simulink model "astron_hw_test_au50_16k_8in"  (R2021a)
settings: Solver=VariableStepDiscrete  StartTime=0.0  StopTime=32000  RelTol=1e-3
undefined symbols (not defined in the file): d0, d1, d2, d3, d4, d5, d6, d7, FFT, sr, Wideband_FFT
libraries: xbsIndex_r4 x1247, casper_library_misc x6, xps_library x1
(part 4 of 17)

== system astron_hw_test_au50_16k_8in/bram_in4 ==
  addr : Inport
  data_in : Inport  Port=2
  we : Inport  Port=3
  Terminator : Terminator
  Terminator1 : Terminator
  Terminator2 : Terminator
  astron_hw_test_au50_16k_8in_bram_in4_addr : xbsIndex_r4/Gateway Out  inherit_from_input=off  hdl_port=on  rows=1  columns=1  UseAsDAC=off  DACChannel='1'  interface=None  automatic_assignment=on  address_offset=hex2dec('00')  intf_name=''  intf_description=''  timing_constraint=None  locs_specified=off  LOCs={'A5','B9','A9','C1','A3','G6','E9','A6','A7','A8','B8','B1','B3','D9','B5','B4','B6','C2'}  io_standard={}  block_type=gatewayout
      settings: infoedit="Gateway out block.  Converts Xilinx fixed point inputs into ouputs of type Simulink integer, double, or fixed point.<P><P>Hardware notes:  In hardware these blocks become top level output ports or are discarded, depending on how they are configured."  sginterface={'Nallatech'=>{'xdspkit'=>{'non_memory_mapped_port'=>'uprev_Shared_BRAM_addr'}},'Xilinx'=>{'jtaghwcosim'=>{'non_memory_mapped_port'=>'uprev_Shared_BRAM_addr'},'xdspkit'=>{'non_memory_mapped_port'=>'uprev_Shared_BRAM_addr'}}}  xl_area=[0, 0, 0, 0, 0, 0, 0]
  astron_hw_test_au50_16k_8in_bram_in4_data_in : xbsIndex_r4/Gateway Out  inherit_from_input=off  hdl_port=on  rows=1  columns=1  UseAsDAC=off  DACChannel='1'  interface=None  automatic_assignment=on  address_offset=hex2dec('00')  intf_name=''  intf_description=''  timing_constraint=None  locs_specified=off  LOCs={'B21','B22','A22','B23','B19','C19','A20','A21','A23','B24','A24','A25','E18','D18','C18','B18'}  io_standard={}  block_type=gatewayout
      settings: infoedit="Gateway out block.  Converts Xilinx fixed point inputs into ouputs of type Simulink integer, double, or fixed point.<P><P>Hardware notes:  In hardware these blocks become top level output ports or are discarded, depending on how they are configured."  sginterface={'Nallatech'=>{'xdspkit'=>{'non_memory_mapped_port'=>'uprev_Shared_BRAM_data_in'}},'Xilinx'=>{'jtaghwcosim'=>{'non_memory_mapped_port'=>'uprev_Shared_BRAM_data_in'},'xdspkit'=>{'non_memory_mapped_port'=>'uprev_Shared_BRAM_data_in'}}}  xl_area=[0, 0, 0, 0, 0, 0, 0]
  astron_hw_test_au50_16k_8in_bram_in4_data_out : xbsIndex_r4/Gateway In  gui_display_data_type=Fixed-point  arith_type=Unsigned  n_bits=32  bin_pt=0  preci_type=Single  exp_width=8  frac_width=24  rows=1  columns=1  quantization=Truncate  overflow=Wrap  period=sample_rate  UseAsADC=off  ADCChannel='1'  interface=None  automatic_assignment=on  address_offset=hex2dec('00')  intf_name=''  intf_description=''  default_value=0  timing_constraint=None  locs_specified=off  LOCs={}  io_standard={}  inherit_from_input=off  hdl_port=on  dbl_ovrd=off  block_type=gatewayin
      settings: xl_area=[0, 0, 0, 0, 0, 0, 0]
  astron_hw_test_au50_16k_8in_bram_in4_we : xbsIndex_r4/Gateway Out  inherit_from_input=off  hdl_port=on  rows=1  columns=1  UseAsDAC=off  DACChannel='1'  interface=None  automatic_assignment=on  address_offset=hex2dec('00')  intf_name=''  intf_description=''  timing_constraint=None  locs_specified=off  LOCs={'A14'}  io_standard={}  block_type=gatewayout
      settings: infoedit="Gateway out block.  Converts Xilinx fixed point inputs into ouputs of type Simulink integer, double, or fixed point.<P><P>Hardware notes:  In hardware these blocks become top level output ports or are discarded, depending on how they are configured."  xl_area=[0, 0, 0, 0, 0, 0, 0]
  calc_add : Subsystem  mask{data_width=32, addr_width=11, sample_rate=sample_rate}
      mask prompts: data_width "data width"; addr_width "address width"; sample_rate "sample rate"
  convert_addr : xbsIndex_r4/Convert  gui_display_data_type=Fixed-point  arith_type=Unsigned  n_bits=addr_width  bin_pt=0  float_type=Single  exp_bits=8  fraction_bits=24  quantization=Truncate  overflow=Wrap  en=off  latency=0  pipeline=off  dbl_ovrd=off  block_type=convert
      settings: xl_area=[0, 0, 0, 0, 0, 0, 0]
  convert_din1 : xbsIndex_r4/Convert  gui_display_data_type=Fixed-point  arith_type=Unsigned  n_bits=32  bin_pt=0  float_type=Single  exp_bits=8  fraction_bits=24  quantization=Truncate  overflow=Wrap  en=off  latency=0  pipeline=off  dbl_ovrd=off  block_type=convert
      settings: xl_area=[0, 0, 0, 0, 0, 0, 0]
  convert_we : xbsIndex_r4/Convert  gui_display_data_type=Fixed-point  arith_type=Unsigned  n_bits=1  bin_pt=0  float_type=Single  exp_bits=8  fraction_bits=24  quantization=Truncate  overflow=Wrap  en=off  latency=0  pipeline=off  dbl_ovrd=off  block_type=convert
      settings: xl_area=[0, 0, 0, 0, 0, 0, 0]
  munge_in : Subsystem  AncestorBlock=casper_library_flow_control/munge  mask(munge){divisions=1, div_size=32, order=[0], arith_type_out=Unsigned, bin_pt_out=0}
      mask prompts: divisions "Number of divisions"; div_size "Division size (bits)"; order "Division packing order"; arith_type_out "Output arithmetic type"; bin_pt_out "Output binary point"
      mask help: Splits an input bus into the specified number of divisions and then recombines them in the order specified (most significant division = 0,least = number divisions-1)
      mask init:
      | munge_init(gcb, ...
      |     'divisions', divisions, ...
      |     'div_size', div_size, ...
      |     'order', order, ...
      |     'arith_type_out', arith_type_out, ...
      |     'bin_pt_out', bin_pt_out);
      settings: AttributesFormatString=|
      | split:32
      | join:0
      | Unsigned [32,0]
      mask TypeOptions arith_type_out: Unsigned | Signed  (2's comp) | Floating-point
  munge_out : Subsystem  AncestorBlock=casper_library_flow_control/munge  mask(munge){divisions=1, div_size=32, order=[0], arith_type_out=Signed  (2's comp), bin_pt_out=0}
      mask prompts: divisions "Number of divisions"; div_size "Division size (bits)"; order "Division packing order"; arith_type_out "Output arithmetic type"; bin_pt_out "Output binary point"
      mask help: Splits an input bus into the specified number of divisions and then recombines them in the order specified (most significant division = 0,least = number divisions-1)
      mask init:
      | munge_init(gcb, ...
      |     'divisions', divisions, ...
      |     'div_size', div_size, ...
      |     'order', order, ...
      |     'arith_type_out', arith_type_out, ...
      |     'bin_pt_out', bin_pt_out);
      settings: AttributesFormatString=|
      | split:32
      | join:0
      | Signed  (2's comp) [32,0]
      mask TypeOptions arith_type_out: Unsigned | Signed  (2's comp) | Floating-point
  sim_mem : Subsystem  mask{arith_type=Signed  (2's comp), addr_width=11, data_width=32, data_bin_pt=0, init_vals=[5372    264   2664  -1583   -209  -8118   2914  -1119   9156  -1791   -682  -1639  -1972  -7418   7738  -6315   6175   2047  -1371  -5922   1133  -4748   4947  -7294    598    694  -2771 -11240  -7297  -1257  10652  -4301    242  -5536  -2316  -5035   -774 -11427   5804  -3502  -2727  -5631   5820  -1336   3152    207   3505  -2899   3712  -5832   -548    499   -949    356   4168  -2711   9110  -1446   -185  -7623   5256   -721  -2371   1834  -3171  -2617  -2004  -5374   8059  -8009   3468  -4248   6229  -5263   7567    392  -2288  -3689   -834   3206   -427   2199   3578  -3080   7720  -4480  -1270  -1827    789  -3782   2421   3593    783   3234  10007  -5331  -3342   3673   3588    706   4326  -4419   -132  -6818   2728  -1544   2912  -6007  -4264  -5624   8559  -4103  -1178   -386   2151  -2551  -1873   3145   1273  -4488  -2723    612   -822  -5199   4364   8473   5041   1818  -1070  -2280   3607  -3180   7444  -4879   6916  -2006   5554  -3584    161   3913   6382   1474   -131  -6736  -3432   1085   3615   -949    406  -3710  10859   -234   3318  -8376   4924   6284  -1230  -6191   2438   1240  -1100  -7300   6874  -1202  -3786   -162  -3936  -1656   3000  -2820   2006  -1797  -4165  -1961   3081  -2189   2194  -5197   5790   2148   1526 -12939   4539   2170   -302  -8231   4511  -4644  -2325  -1395  -2217  -5029   -259    343   4026  11402   9172    170   3063   7245   2744   2974   -116   2113   5449   -744   1639  -8436   2860   7361   -750  -2950   5828   4070   4301  -3510  -3373    239   6919   5964   -550  -3159   2494  -2931   3776  -2781  -1672    540  11327   3666   7426  -7651   2220  -4925   5619   -307   7830  -8896   3110  -7112   8450   -647   5009  -4269   1593  -3851   1861    757   3866    346    -32  -6926  -2968   -124   2070  -6109  -1641 -12060  -1216  -2148  -3305   3381  -8059   -991   5600    890   -676  -8576   6527  -2235   6327  -1480  -2544  -3362  -3643    176  -2266  -4719   5604   1756  10810  -3044    204  -3243   5925   9325  11724   -278    787   1475    253  -2705   1253  -6883   4739    492   2583   4196   -702    919   4520   2806   -557   -919   6700    429   1604  -5668   5381  -5403  -4298   3048   1914   1868   -221  -1599   1680   -408   4556  -2677    531  -3197  10488  -1424   7178  -8210   1200 -10397  -1686  -6020   7446  -3039   6340     44  -2611   6013    813  -6576  -5465   2793   7907  -2877   2051  -3612   2879   -858    -20   -343   5516  -3239    276  -6001   7400  -4314  -1066  -1650   2581  -7150   7801  -5366   2259  -3747  -1802  -3143  -4562   -217   2213  -3598    380   1819    459 -11485   1496   3375   5261  -4536   2628  -4517   2812  -2382   2159   2459   1499   -603  -3458  -6213  -1555  -9169  -7572   3950   1325   -737    293    352   5860  -4078   3580  -3457  -2420   3374   5013   2542   1417  -2648    639   2635  -1587  -7108   1615  -6830  -1268  -3826  -7575  -3513   9379  -1148  -1833  -4949    799  -1823     85   2797   4700   1680   5387  -8986  -2486    672   4069  -2791   4382  -4512  -5528  -4235  -7648  -8826   5712   2253    420   4054  -1483  -3200  -1126  -3146  -4911  -8683  -6029    797   6606  -7828  -3268    594  -4858   6717   -412   2169   4283  -2812   1675   2976    658    -72   3034  -4769   3257   1926  -4680  -2421   9476  -1206   2513   4604   7309  -3175  -1675   -869   4580   3774   6399    313  -1949   -886  -2670   3019   5781  -4535   2075   2994    445  -7441   1585  -5266   2359  -7332   2614    880   1385  -2791    426  -2620   2687   1016   3193   1554   3871  -5678   3982    709   3608   6326   6781  -2259   7111  -3020    309   -524  -5932   5448   1493  -2473    647  -3940  -6107    978   2317   3384   6445   2742  -1063  -1003   3804  -2802  -9392    840    253  -2545  -1521    886   -283  -5068   3741   1149   5145  -6183   -177  -1297   6951  -1706   5403  -2825  -1015   -519  -5040 -13537  -2391  -4401  11546  -1835   3685  -5829  -2937 -12387   3257    296   5361  -2724   3034  -4443   -152   4231   3085 ...(+10338 chars)], sample_rate=1, csp_latency=1}
      mask prompts: arith_type "Output Data Type"; addr_width "Address width"; data_width "Data width"; data_bin_pt "Data Binary Point"; init_vals "Initial values"; sample_rate "Sample rate"; csp_latency "Latency"
      mask init:
      | % set_param([gcb, '/data_to_xilinx'], 'arith_type', arith_type)
      | % set_param([gcb, '/data_to_xilinx'], 'n_bits', get_param(gcb, 'data_width'))
      mask TypeOptions arith_type: Unsigned | Signed  (2's comp)
      mask TypeOptions data_width: 8 | 16 | 32 | 64 | 128
  data_out : Outport  VectorParamsAs1DForOutWhenUnconnected=off
  wires:
  munge_out/1(dout) -> data_out/1
  sim_mem/1(data_out) -> astron_hw_test_au50_16k_8in_bram_in4_data_out/1
  astron_hw_test_au50_16k_8in_bram_in4_data_out/1 -> munge_out/1(din)
  convert_addr/1 -> astron_hw_test_au50_16k_8in_bram_in4_addr/1
  convert_din1/1 -> astron_hw_test_au50_16k_8in_bram_in4_data_in/1
  data_in/1 -> munge_in/1(din)
  calc_add/1(out) -> convert_addr/1
  astron_hw_test_au50_16k_8in_bram_in4_we/1 -> Terminator2/1
  astron_hw_test_au50_16k_8in_bram_in4_data_in/1 -> Terminator1/1
  astron_hw_test_au50_16k_8in_bram_in4_addr/1 -> Terminator/1
  convert_we/1 -> astron_hw_test_au50_16k_8in_bram_in4_we/1
  addr/1 -> sim_mem/1(addr), calc_add/1(in)
  we/1 -> sim_mem/3(we), convert_we/1
  munge_in/1(dout) -> sim_mem/2(data), convert_din1/1

== system astron_hw_test_au50_16k_8in/bram_in5 ==
  addr : Inport
  data_in : Inport  Port=2
  we : Inport  Port=3
  Terminator : Terminator
  Terminator1 : Terminator
  Terminator2 : Terminator
  astron_hw_test_au50_16k_8in_bram_in5_addr : xbsIndex_r4/Gateway Out  inherit_from_input=off  hdl_port=on  rows=1  columns=1  UseAsDAC=off  DACChannel='1'  interface=None  automatic_assignment=on  address_offset=hex2dec('00')  intf_name=''  intf_description=''  timing_constraint=None  locs_specified=off  LOCs={'A5','B9','A9','C1','A3','G6','E9','A6','A7','A8','B8','B1','B3','D9','B5','B4','B6','C2'}  io_standard={}  block_type=gatewayout
      settings: infoedit="Gateway out block.  Converts Xilinx fixed point inputs into ouputs of type Simulink integer, double, or fixed point.<P><P>Hardware notes:  In hardware these blocks become top level output ports or are discarded, depending on how they are configured."  sginterface={'Nallatech'=>{'xdspkit'=>{'non_memory_mapped_port'=>'uprev_Shared_BRAM_addr'}},'Xilinx'=>{'jtaghwcosim'=>{'non_memory_mapped_port'=>'uprev_Shared_BRAM_addr'},'xdspkit'=>{'non_memory_mapped_port'=>'uprev_Shared_BRAM_addr'}}}  xl_area=[0, 0, 0, 0, 0, 0, 0]
  astron_hw_test_au50_16k_8in_bram_in5_data_in : xbsIndex_r4/Gateway Out  inherit_from_input=off  hdl_port=on  rows=1  columns=1  UseAsDAC=off  DACChannel='1'  interface=None  automatic_assignment=on  address_offset=hex2dec('00')  intf_name=''  intf_description=''  timing_constraint=None  locs_specified=off  LOCs={'B21','B22','A22','B23','B19','C19','A20','A21','A23','B24','A24','A25','E18','D18','C18','B18'}  io_standard={}  block_type=gatewayout
      settings: infoedit="Gateway out block.  Converts Xilinx fixed point inputs into ouputs of type Simulink integer, double, or fixed point.<P><P>Hardware notes:  In hardware these blocks become top level output ports or are discarded, depending on how they are configured."  sginterface={'Nallatech'=>{'xdspkit'=>{'non_memory_mapped_port'=>'uprev_Shared_BRAM_data_in'}},'Xilinx'=>{'jtaghwcosim'=>{'non_memory_mapped_port'=>'uprev_Shared_BRAM_data_in'},'xdspkit'=>{'non_memory_mapped_port'=>'uprev_Shared_BRAM_data_in'}}}  xl_area=[0, 0, 0, 0, 0, 0, 0]
  astron_hw_test_au50_16k_8in_bram_in5_data_out : xbsIndex_r4/Gateway In  gui_display_data_type=Fixed-point  arith_type=Unsigned  n_bits=32  bin_pt=0  preci_type=Single  exp_width=8  frac_width=24  rows=1  columns=1  quantization=Truncate  overflow=Wrap  period=sample_rate  UseAsADC=off  ADCChannel='1'  interface=None  automatic_assignment=on  address_offset=hex2dec('00')  intf_name=''  intf_description=''  default_value=0  timing_constraint=None  locs_specified=off  LOCs={}  io_standard={}  inherit_from_input=off  hdl_port=on  dbl_ovrd=off  block_type=gatewayin
      settings: xl_area=[0, 0, 0, 0, 0, 0, 0]
  astron_hw_test_au50_16k_8in_bram_in5_we : xbsIndex_r4/Gateway Out  inherit_from_input=off  hdl_port=on  rows=1  columns=1  UseAsDAC=off  DACChannel='1'  interface=None  automatic_assignment=on  address_offset=hex2dec('00')  intf_name=''  intf_description=''  timing_constraint=None  locs_specified=off  LOCs={'A14'}  io_standard={}  block_type=gatewayout
      settings: infoedit="Gateway out block.  Converts Xilinx fixed point inputs into ouputs of type Simulink integer, double, or fixed point.<P><P>Hardware notes:  In hardware these blocks become top level output ports or are discarded, depending on how they are configured."  xl_area=[0, 0, 0, 0, 0, 0, 0]
  calc_add : Subsystem  mask{data_width=32, addr_width=11, sample_rate=sample_rate}
      mask prompts: data_width "data width"; addr_width "address width"; sample_rate "sample rate"
  convert_addr : xbsIndex_r4/Convert  gui_display_data_type=Fixed-point  arith_type=Unsigned  n_bits=addr_width  bin_pt=0  float_type=Single  exp_bits=8  fraction_bits=24  quantization=Truncate  overflow=Wrap  en=off  latency=0  pipeline=off  dbl_ovrd=off  block_type=convert
      settings: xl_area=[0, 0, 0, 0, 0, 0, 0]
  convert_din1 : xbsIndex_r4/Convert  gui_display_data_type=Fixed-point  arith_type=Unsigned  n_bits=32  bin_pt=0  float_type=Single  exp_bits=8  fraction_bits=24  quantization=Truncate  overflow=Wrap  en=off  latency=0  pipeline=off  dbl_ovrd=off  block_type=convert
      settings: xl_area=[0, 0, 0, 0, 0, 0, 0]
  convert_we : xbsIndex_r4/Convert  gui_display_data_type=Fixed-point  arith_type=Unsigned  n_bits=1  bin_pt=0  float_type=Single  exp_bits=8  fraction_bits=24  quantization=Truncate  overflow=Wrap  en=off  latency=0  pipeline=off  dbl_ovrd=off  block_type=convert
      settings: xl_area=[0, 0, 0, 0, 0, 0, 0]
  munge_in : Subsystem  AncestorBlock=casper_library_flow_control/munge  mask(munge){divisions=1, div_size=32, order=[0], arith_type_out=Unsigned, bin_pt_out=0}
      mask prompts: divisions "Number of divisions"; div_size "Division size (bits)"; order "Division packing order"; arith_type_out "Output arithmetic type"; bin_pt_out "Output binary point"
      mask help: Splits an input bus into the specified number of divisions and then recombines them in the order specified (most significant division = 0,least = number divisions-1)
      mask init:
      | munge_init(gcb, ...
      |     'divisions', divisions, ...
      |     'div_size', div_size, ...
      |     'order', order, ...
      |     'arith_type_out', arith_type_out, ...
      |     'bin_pt_out', bin_pt_out);
      settings: AttributesFormatString=|
      | split:32
      | join:0
      | Unsigned [32,0]
      mask TypeOptions arith_type_out: Unsigned | Signed  (2's comp) | Floating-point
  munge_out : Subsystem  AncestorBlock=casper_library_flow_control/munge  mask(munge){divisions=1, div_size=32, order=[0], arith_type_out=Signed  (2's comp), bin_pt_out=0}
      mask prompts: divisions "Number of divisions"; div_size "Division size (bits)"; order "Division packing order"; arith_type_out "Output arithmetic type"; bin_pt_out "Output binary point"
      mask help: Splits an input bus into the specified number of divisions and then recombines them in the order specified (most significant division = 0,least = number divisions-1)
      mask init:
      | munge_init(gcb, ...
      |     'divisions', divisions, ...
      |     'div_size', div_size, ...
      |     'order', order, ...
      |     'arith_type_out', arith_type_out, ...
      |     'bin_pt_out', bin_pt_out);
      settings: AttributesFormatString=|
      | split:32
      | join:0
      | Signed  (2's comp) [32,0]
      mask TypeOptions arith_type_out: Unsigned | Signed  (2's comp) | Floating-point
  sim_mem : Subsystem  mask{arith_type=Signed  (2's comp), addr_width=11, data_width=32, data_bin_pt=0, init_vals=[3085   4112   3544   1678  -1800    776   3294   1264  -1429  -4034   1131  -4445  -4928    183  12343  -5388    845  -1061   2787   2474   3321  -5924   9147   2948  -1169  -7781  -4502  -4890    976   1720   2508  -8281   4106   3611    885  -3616   5662 -12635   3325   -343   3434   3105   2550   3008   -201  -6122   3077   4239  -1309   -698  -1645  -9855   3889   3243   -135   2950  -3051    655   5749   2697  -6099  -6840   -804  -8880   4783  -1844   5694   -857  -2457  -2128   7001   -273   6624  -1099  -1959  -6239   1805    854  11189  -3682   -313  -1304  -1204   3537   1658  -2051   1394    425   1804  -2617   3829  -6720   5201  -4609  -8211   -235  -5823  -1330  -3121   4064   1860  -5034  -3714   5586   -271   1706   5634  -9076   4269   1067   -684   1929   8778  -3811    556  -5552   2807   3804   2813   7339   5371   -814    359  -4198   3079   2550  -2554   1018    462  -8743   4298  -4165  -7870   4693   -725  -3794   1675   -303   -530  -2828   8909   -265   4757  -5900  -2683     49  -2186  -9215   -975  -2675  -1505  -1568   1443  -6865  -2485  -7290  -6915  -9449   2648  -5374   1271   1444   5601   2379   7764   -967    303   -341  -9376  -1648   8819    -39  12043  -3198  -2472  -9660   6711  -3417   -769    820  -2005   2484  -9339   -279   4766    817    126    772   2056  -4808   3274  -7998   6813  -1749   3845   3291  -1914   1824  -3279  -5271   7212   -109  -2123  -2250   1800  -4350   4172   3743    903  -3989    709  -1685   3221  -2913   1792  -4029  10766   2275   1807    -64   4351    182   5543  -5001  -2146   3872   1319  -2628   4274   3856   1211  -1088   3958   1153   5056  -2594    860   5101  -1864  -5845   4257  -2147   1901 -11590  -2242   3948   1163  -2475   -674  -4259  -4987   4277   4506   1237   5321  -3272   7910  -1396  -1514   2153   8800  -7213   6032  -2137  -4624  -1098   8720   3800   2834  -4352   2706 -10261  -1053   2194  -1662  -2273   9675  -2289  -2089  -3522   3670   4494   2300  -9828   -279  -9950    279  -6076   -259   6198  -1182  -1323  -1507  -4354   5644  -1634   5775    284   1153   1884   4174  -4194   3955   -477  -1044  -4851  -4658  -6393   6373  -1850   -412  -2720  -3705  -6353   3706   1553   2360   5349  -1510  -8544   4141  -2035  -1792   -978   1685  -5478   2606  -6096   4780  -6151   3319  -7017   5258   6125   2397  -3572   2856   2742   2686    107   2700   -374   4054  -4846  10685  -4792   2948  -6392   -563  -1043   7529   2795  -5968  -2384   9941   1009    300   7811  -1658    237  -1416  -3846   5364   5750   -796   4908   4365  -4727  -2428   1010   3218  -8480   2860  -6992   6717  -6058   2848  -3346   1318  -2278   4113  -3080   3586  -8431  -3372  -2742   3411   1290   3316  -5467   3053   1799  12208   2360    229  -5859   4015  -2602   5050   6682   3552   1972   -636    720   4094  -3218   1781  -2651  -4157    835    605  -2362   3549  -1123   -210    457   -613  -4279   -522    231  -5218  -6897   3774  -4294  -4372  -1816   4175 -10615   4284  -5381   3638   2304   2987  -8007  -1606   2359    760   -354  -1504  -6605   -141     39   5432  -1104   4484  -6737   2913  -7381  -4432    286   3679   4945    159   5156    162   2543   5147   1268  -2721   1889  -1830   2910   3864  -2275    430    178    129  -7093   9818  -3158   4019   -600  -1348   1005  -1450  -2630   3013   -906  -2948  -8606    802   -542   -109  -3665   4599   2619    112   1134   2825  -7297   7525   -647  -2595  -7671    141   1253   1800  -8781   3734  -1271  -2819    348   4057    399   3556  -4514   4240   3302  -1897   7370  -8605   3006   6744  -2909  10787  -3404   6731  -5888  -2217  -4857   1034   1838    769  -2156   1593   1666    603   5227  -1252  -2168   5348 -10404  -8384   7448   3201  -7482   3142  -6127  -2482   2003   4428   1787   5299   3487   1227   -635   8787   1664   2507 -10276   4317   -316    458  -5642   1201  -5740   6855  -8190   4095  -3351  -1775    129   6168  -3735  -2430  -4103  -2129   -170   -519    707  -5235 ...(+10337 chars)], sample_rate=1, csp_latency=1}
      mask prompts: arith_type "Output Data Type"; addr_width "Address width"; data_width "Data width"; data_bin_pt "Data Binary Point"; init_vals "Initial values"; sample_rate "Sample rate"; csp_latency "Latency"
      mask init:
      | % set_param([gcb, '/data_to_xilinx'], 'arith_type', arith_type)
      | % set_param([gcb, '/data_to_xilinx'], 'n_bits', get_param(gcb, 'data_width'))
      mask TypeOptions arith_type: Unsigned | Signed  (2's comp)
      mask TypeOptions data_width: 8 | 16 | 32 | 64 | 128
  data_out : Outport  VectorParamsAs1DForOutWhenUnconnected=off
  wires:
  munge_out/1(dout) -> data_out/1
  sim_mem/1(data_out) -> astron_hw_test_au50_16k_8in_bram_in5_data_out/1
  astron_hw_test_au50_16k_8in_bram_in5_data_out/1 -> munge_out/1(din)
  convert_addr/1 -> astron_hw_test_au50_16k_8in_bram_in5_addr/1
  convert_din1/1 -> astron_hw_test_au50_16k_8in_bram_in5_data_in/1
  data_in/1 -> munge_in/1(din)
  calc_add/1(out) -> convert_addr/1
  astron_hw_test_au50_16k_8in_bram_in5_we/1 -> Terminator2/1
  astron_hw_test_au50_16k_8in_bram_in5_data_in/1 -> Terminator1/1
  astron_hw_test_au50_16k_8in_bram_in5_addr/1 -> Terminator/1
  convert_we/1 -> astron_hw_test_au50_16k_8in_bram_in5_we/1
  addr/1 -> sim_mem/1(addr), calc_add/1(in)
  we/1 -> sim_mem/3(we), convert_we/1
  munge_in/1(dout) -> sim_mem/2(data), convert_din1/1
